simulink model "SIM_Overview"  (R2020b)
settings: Solver=FixedStepAuto  StartTime=0.0  StopTime=params.time.stop  FixedStep=1  RelTol=1e-3
PreLoadFcn:
  | run('sim_initial_values.m')
values from neighbouring files (symbols this model uses):
  data = get_scenario(1)    [sim_initial_values.m]
  solar = get_solar_from_file(data.Date(1),data.Date(end))    [sim_initial_values.m]
undefined symbols (not defined in the file or in its folder): days, params, seconds
libraries: mylib x5
settings Model: Creator=janluca  LastModifiedBy=janluca
settings DataIOCC: LimitDataPoints=on  MaxDataPoints=1

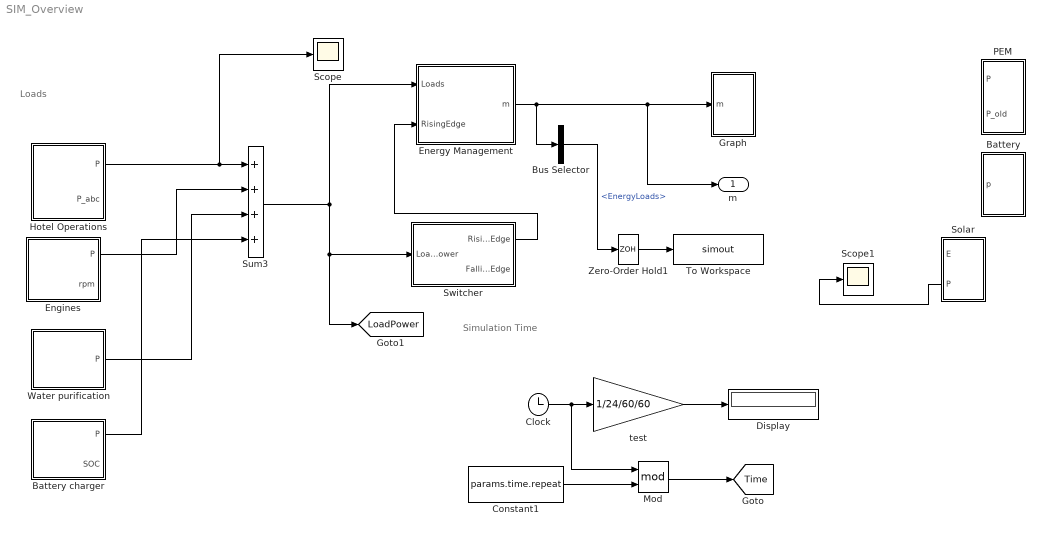
== system SIM_Overview ==
  note: Loads
  note: Simulation Time
  Battery : Subsystem
  Battery charger : Subsystem
  Bus Selector : BusSelector  OutputSignals=EnergyLoads
  Clock : Clock
      settings: Decimation=60000
  Constant1 : Constant  Value=params.time.repeat
  Display : Display
  Energy Management : Subsystem
  Engines : Subsystem
      mask Display: image('/Users/janluca/Projects/git/Masterthesis/MATLAB/icons/motor2.jpg'); % Use "Edit Image" on toolstrip to change.
  Graph : Subsystem
  Hotel Operations : Subsystem
      mask Display: image('/Users/janluca/Projects/git/Masterthesis/MATLAB/icons/bar.jpg'); % Use "Edit Image" on toolstrip to change.
  Mod : Math  Operator=mod  OutMin=[1]  OutMax=[3600]  SaturateOnIntegerOverflow=on
  PEM : Subsystem
  Scope : Scope
  Scope1 : Scope
  Solar : Subsystem
  Sum3 : Sum  Inputs=4
  Switcher : Subsystem
  To Workspace : ToWorkspace  VariableName=simout  SaveFormat=Timeseries  SampleTime=-1
  Water purification : Subsystem
      mask Display: image('/Users/janluca/Projects/git/Masterthesis/MATLAB/icons/wasserhahn.jpg'); % Use "Edit Image" on toolstrip to change.
  Zero-Order Hold1 : ZeroOrderHold  SampleTime=seconds(days(1))
  test : Gain  Gain=1/24/60/60
  m : Outport
  tag scope: LoadPower=global, Time=global
  wires:
  test/1 -> Display/1
  Constant1/1 -> Mod/2
  Mod/1 -> [Time]
  Clock/1 -> test/1, Mod/1
  Switcher/1(RisingEdge) -> Energy Management/2(RisingEdge)
  Energy Management/1(m) -> Bus Selector/1, m/1, Graph/1(m)
  Hotel Operations/1(P) -> Scope/1, Sum3/1
  Engines/1(P) -> Sum3/2
  Water purification/1(P) -> Sum3/3
  Battery charger/1(P) -> Sum3/4
  Sum3/1 -> [LoadPower], Switcher/1(LoadPower), Energy Management/1(Loads)
  Solar/2(P) -> Scope1/1
  Zero-Order Hold1/1 -> To Workspace/1
  Bus Selector/1 -> Zero-Order Hold1/1  "<EnergyLoads>"

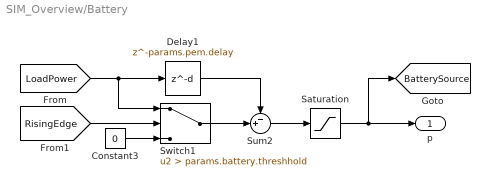
== system SIM_Overview/Battery ==
  Constant3 : Constant  Value=0
  Delay1 : Delay  DelayLength=params.pem.delay
  Saturation : Saturate  UpperLimit=params.battery.power  LowerLimit=0
  Sum2 : Sum  Inputs=-+|
  Switch1 : Switch  Criteria=u2 > Threshold  Threshold=params.battery.threshhold
  p : Outport
  tag scope: BatterySource=global
  wires:
  Constant3/1 -> Switch1/3
  Delay1/1 -> Sum2/1
  [LoadPower] -> Switch1/1, Delay1/1
  Sum2/1 -> Saturation/1
  Saturation/1 -> [BatterySource], p/1
  Switch1/1 -> Sum2/2
  [RisingEdge] -> Switch1/2

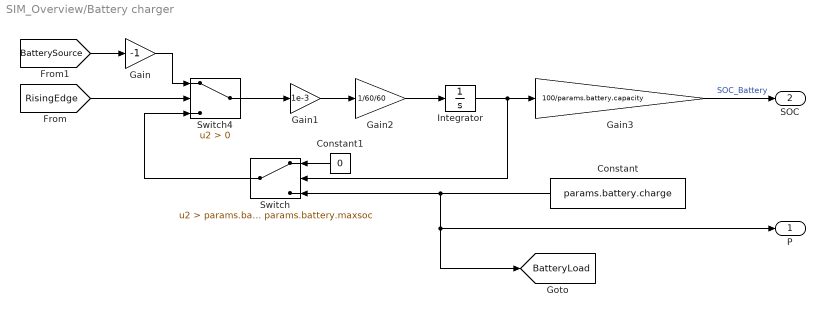
== system SIM_Overview/Battery charger ==
  Constant : Constant  Value=params.battery.charge
  Constant1 : Constant  Value=0
  Gain : Gain  Gain=-1
  Gain1 : Gain  Gain=1e-3
  Gain2 : Gain  Gain=1/60/60
  Gain3 : Gain  Gain=100/params.battery.capacity
  Integrator : Integrator  InitialCondition=params.battery.capacity * params.battery.initsoc
  Switch : Switch  Criteria=u2 > Threshold  Threshold=params.battery.capacity * params.battery.maxsoc
  Switch4 : Switch  Criteria=u2 > Threshold
  P : Outport
  SOC : Outport  Port=2
  tag scope: BatteryLoad=global
  wires:
  Gain1/1 -> Gain2/1
  Constant/1 -> P/1, [BatteryLoad], Switch/3
  Integrator/1 -> Switch/2, Gain3/1
  Gain/1 -> Switch4/1
  Gain2/1 -> Integrator/1
  Constant1/1 -> Switch/1
  Switch4/1 -> Gain1/1
  Switch/1 -> Switch4/3
  Gain3/1 -> SOC/1  "SOC_Battery"
  [RisingEdge] -> Switch4/2
  [BatterySource] -> Gain/1

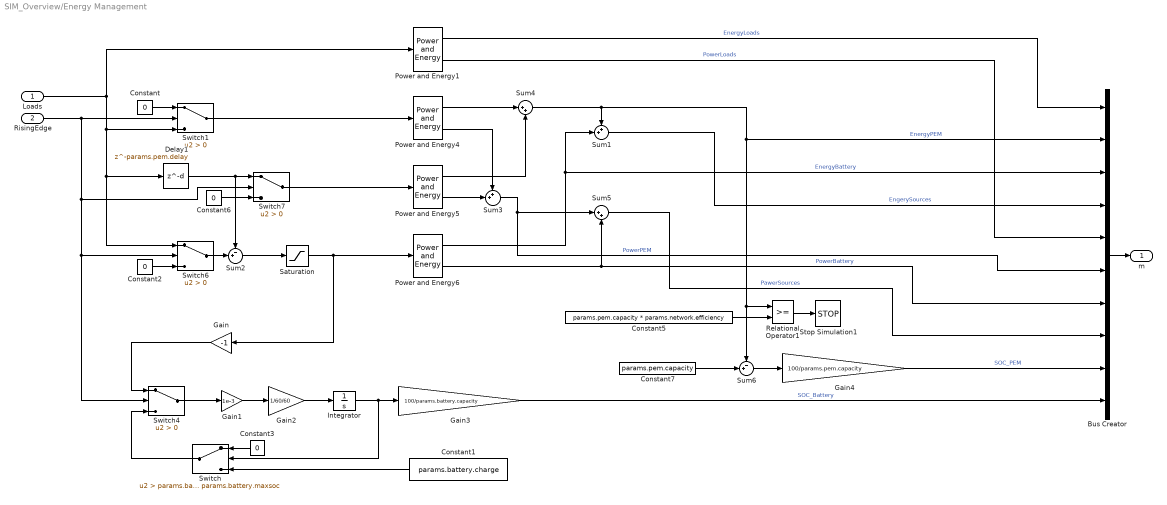
== system SIM_Overview/Energy Management ==
  Loads : Inport
  RisingEdge : Inport  Port=2
  Bus Creator : BusCreator  Inputs=10
  Constant{,2..3,6} (4 alike) : Constant  Value=0
  Constant1 : Constant  Value=params.battery.charge
  Constant5 : Constant  Value=params.pem.capacity * params.network.efficiency
  Constant7 : Constant  Value=params.pem.capacity
  Delay1 : Delay  DelayLength=params.pem.delay
  Gain : Gain  Gain=-1
  Gain1 : Gain  Gain=1e-3
  Gain2 : Gain  Gain=1/60/60
  Gain3 : Gain  Gain=100/params.battery.capacity
  Gain4 : Gain  Gain=100/params.pem.capacity
  Integrator : Integrator  InitialCondition=params.battery.capacity * params.battery.initsoc
  Power and Energy{1,4..6} (4 alike) : mylib/Power and Energy  SystemSampleTime=-1  VariantActivationTime=update diagram  Latency=0  AutoFrameSizeCalculation=off
  Relational Operator1 : RelationalOperator  OutDataTypeStr=boolean  RndMeth=Simplest
  Saturation : Saturate  UpperLimit=inf  LowerLimit=0
  Stop Simulation1 : Stop
  Sum1 : Sum  Inputs=++|
  Sum2 : Sum  Inputs=-+|
  Sum3 : Sum  Inputs=++|
  Sum4 : Sum  Inputs=|++
  Sum5 : Sum  Inputs=|++
  Sum6 : Sum  Inputs=-+|
  Switch : Switch  Criteria=u2 > Threshold  Threshold=params.battery.capacity * params.battery.maxsoc
  Switch{1,4,6..7} (4 alike) : Switch  Criteria=u2 > Threshold
  m : Outport
  wires:
  Loads/1 -> Switch6/1, Delay1/1, Switch1/3, Power and Energy1/1
  Constant/1 -> Switch1/1
  Constant2/1 -> Switch6/3
  Switch1/1 -> Power and Energy4/1
  Switch6/1 -> Sum2/2
  Sum2/1 -> Saturation/1
  Delay1/1 -> Sum2/1, Switch7/1
  Switch7/1 -> Power and Energy5/1
  Constant6/1 -> Switch7/3
  Power and Energy4/1 -> Sum4/1
  Power and Energy5/1 -> Sum4/2
  Sum4/1 -> Sum1/1, Bus Creator/2, Relational Operator1/1, Sum6/1  "EnergyPEM"
  Constant5/1 -> Relational Operator1/2
  Relational Operator1/1 -> Stop Simulation1/1
  Power and Energy6/1 -> Sum1/2, Bus Creator/3  "EnergyBattery"
  Sum1/1 -> Bus Creator/4  "EngerySources"
  Power and Energy5/2 -> Sum3/2
  Power and Energy4/2 -> Sum3/1
  Sum3/1 -> Bus Creator/6, Sum5/1  "PowerPEM"
  Sum5/1 -> Bus Creator/8  "PawerSources"
  Power and Energy6/2 -> Sum5/2, Bus Creator/7  "PowerBattery"
  Sum6/1 -> Gain4/1
  Constant7/1 -> Sum6/2
  Power and Energy1/1 -> Bus Creator/1  "EnergyLoads"
  Power and Energy1/2 -> Bus Creator/5  "PowerLoads"
  Gain4/1 -> Bus Creator/9  "SOC_PEM"
  Bus Creator/1 -> m/1
  Gain3/1 -> Bus Creator/10  "SOC_Battery"
  Gain2/1 -> Integrator/1
  Constant1/1 -> Switch/3
  Switch/1 -> Switch4/3
  Constant3/1 -> Switch/1
  Switch4/1 -> Gain1/1
  Gain/1 -> Switch4/1
  Gain1/1 -> Gain2/1
  RisingEdge/1 -> Switch4/2, Switch6/2, Switch7/2, Switch1/2
  Integrator/1 -> Switch/2, Gain3/1
  Saturation/1 -> Gain/1, Power and Energy6/1

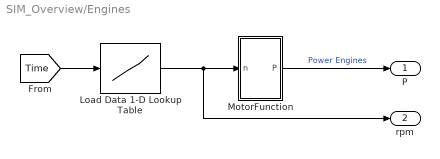
== system SIM_Overview/Engines ==
  Load Data 1-D Lookup Table : Lookup_n-D  NumberOfTableDimensions=1  BreakpointsForDimension1=data.time  BeginIndexSearchUsingPreviousIndexResult=on  Table=data.rpm  InternalRulePriority=Speed  RndMeth=Simplest  InputSameDT=on
  MotorFunction : Subsystem
  P : Outport
  rpm : Outport  Port=2
  wires:
  Load Data 1-D Lookup Table/1 -> rpm/1, MotorFunction/1(n)
  MotorFunction/1(P) -> P/1  "Power Engines"
  [Time] -> Load Data 1-D Lookup Table/1

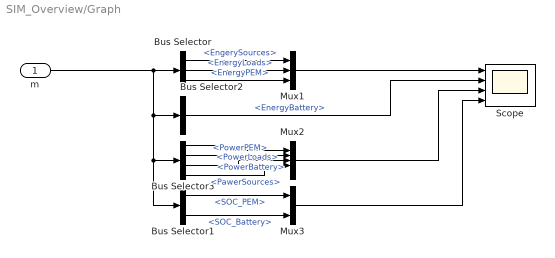
== system SIM_Overview/Graph ==
  m : Inport
  Bus Selector : BusSelector  OutputSignals=EngerySources,EnergyLoads,EnergyPEM
  Bus Selector1 : BusSelector  OutputSignals=SOC_PEM,SOC_Battery
  Bus Selector2 : BusSelector  OutputSignals=EnergyBattery
  Bus Selector3 : BusSelector  OutputSignals=PowerLoads,PowerPEM,PowerBattery,PawerSources
  Mux1 : Mux  Inputs=3
  Mux2 : Mux  Inputs=5
  Mux3 : Mux  Inputs=2
  Scope : Scope  NumInputPorts=4
  wires:
  m/1 -> Bus Selector2/1, Bus Selector3/1, Bus Selector1/1, Bus Selector/1
  Mux1/1 -> Scope/1
  Bus Selector2/1 -> Scope/2  "<EnergyBattery>"
  Bus Selector/2 -> Mux1/2  "<EnergyLoads>"
  Bus Selector3/4 -> Mux2/4  "<PawerSources>"
  Mux2/1 -> Scope/3
  Bus Selector3/3 -> Mux2/3  "<PowerBattery>"
  Bus Selector1/1 -> Mux3/1  "<SOC_PEM>"
  Bus Selector/3 -> Mux1/3  "<EnergyPEM>"
  Bus Selector3/2 -> Mux2/2  "<PowerPEM>"
  Bus Selector1/2 -> Mux3/2  "<SOC_Battery>"
  Mux3/1 -> Scope/4
  Bus Selector/1 -> Mux1/1  "<EngerySources>"
  Bus Selector3/1 -> Mux2/1  "<PowerLoads>"

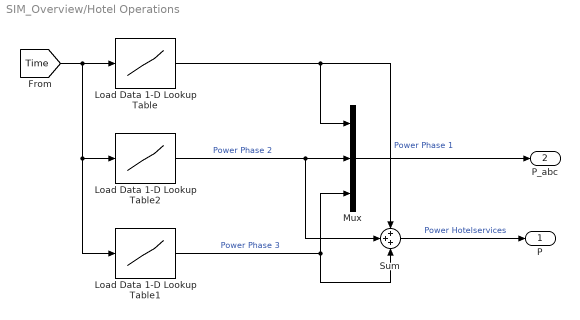
== system SIM_Overview/Hotel Operations ==
  Load Data 1-D Lookup Table : Lookup_n-D  NumberOfTableDimensions=1  BreakpointsForDimension1=data.time  BeginIndexSearchUsingPreviousIndexResult=on  Table=data.P11min  InternalRulePriority=Speed  RndMeth=Simplest  InputSameDT=on
  Load Data 1-D Lookup Table1 : Lookup_n-D  NumberOfTableDimensions=1  BreakpointsForDimension1=data.time  BeginIndexSearchUsingPreviousIndexResult=on  Table=data.P31min  InternalRulePriority=Speed  RndMeth=Simplest  InputSameDT=on
  Load Data 1-D Lookup Table2 : Lookup_n-D  NumberOfTableDimensions=1  BreakpointsForDimension1=data.time  BeginIndexSearchUsingPreviousIndexResult=on  Table=data.P21min  InternalRulePriority=Speed  RndMeth=Simplest  InputSameDT=on
  Mux : Mux  Inputs=3
  Sum : Sum  Inputs=+++
  P : Outport
  P_abc : Outport  Port=2
  wires:
  Load Data 1-D Lookup Table/1 -> Mux/1, Sum/1  "Power Phase 1"
  Load Data 1-D Lookup Table2/1 -> Sum/2, Mux/2  "Power Phase 2"
  Load Data 1-D Lookup Table1/1 -> Sum/3, Mux/3  "Power Phase 3"
  Mux/1 -> P_abc/1
  [Time] -> Load Data 1-D Lookup Table1/1, Load Data 1-D Lookup Table2/1, Load Data 1-D Lookup Table/1
  Sum/1 -> P/1  "Power Hotelservices"

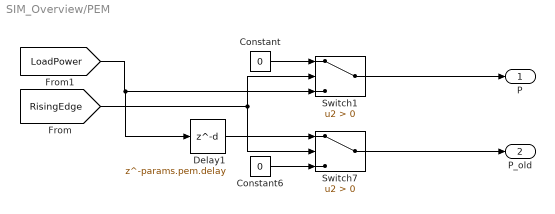
== system SIM_Overview/PEM ==
  Constant : Constant  Value=0
  Constant6 : Constant  Value=0
  Delay1 : Delay  DelayLength=params.pem.delay
  Switch1 : Switch  Criteria=u2 > Threshold
  Switch7 : Switch  Criteria=u2 > Threshold
  P : Outport
  P_old : Outport  Port=2
  wires:
  Switch1/1 -> P/1
  [RisingEdge] -> Switch1/2, Switch7/2
  Constant6/1 -> Switch7/3
  [LoadPower] -> Delay1/1, Switch1/3
  Delay1/1 -> Switch7/1
  Constant/1 -> Switch1/1
  Switch7/1 -> P_old/1

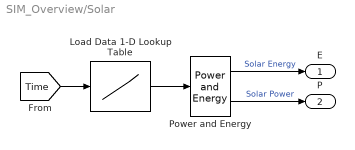
== system SIM_Overview/Solar ==
  Load Data 1-D Lookup Table : Lookup_n-D  NumberOfTableDimensions=1  BreakpointsForDimension1=solar.time  BeginIndexSearchUsingPreviousIndexResult=on  Table=solar.power  InternalRulePriority=Speed  RndMeth=Simplest  InputSameDT=on
  Power and Energy : mylib/Power and Energy  SystemSampleTime=-1  VariantActivationTime=update diagram  Latency=0  AutoFrameSizeCalculation=off
  E : Outport
  P : Outport  Port=2
  wires:
  Power and Energy/2 -> P/1  "Solar Power"
  Power and Energy/1 -> E/1  "Solar Energy"
  [Time] -> Load Data 1-D Lookup Table/1
  Load Data 1-D Lookup Table/1 -> Power and Energy/1

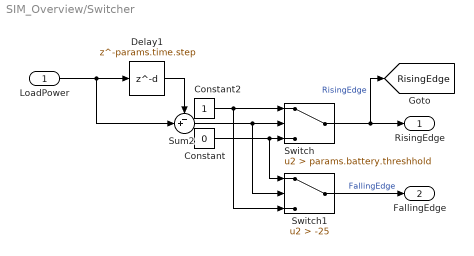
== system SIM_Overview/Switcher ==
  LoadPower : Inport
  Constant : Constant  Value=0
  Constant2 : Constant
  Delay1 : Delay  DelayLength=params.time.step
  Sum2 : Sum  Inputs=-+|
  Switch : Switch  Criteria=u2 > Threshold  Threshold=params.battery.threshhold
  Switch1 : Switch  Criteria=u2 > Threshold  Threshold=-25
  RisingEdge : Outport
  FallingEdge : Outport  Port=2
  tag scope: RisingEdge=global
  wires:
  Switch/1 -> [RisingEdge], RisingEdge/1  "RisingEdge"
  LoadPower/1 -> Sum2/2, Delay1/1
  Delay1/1 -> Sum2/1
  Constant/1 -> Switch1/1, Switch/3
  Switch1/1 -> FallingEdge/1  "FallingEdge"
  Constant2/1 -> Switch/1, Switch1/3
  Sum2/1 -> Switch/2, Switch1/2

== system SIM_Overview/Water purification ==
  Constant3 : Constant  Value=0.5e3
  P : Outport
  wires:
  Constant3/1 -> P/1  "Power water purification"

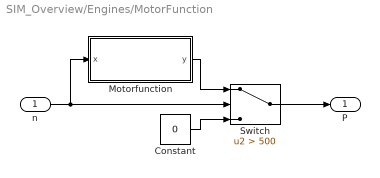
== system SIM_Overview/Engines/MotorFunction ==
  n : Inport
  Constant : Constant  Value=0
  Motorfunction : Subsystem  TreatAsAtomicUnit=on
  Switch : Switch  Criteria=u2 > Threshold  Threshold=500
  P : Outport
  wires:
  n/1 -> Switch/2, Motorfunction/1(x)
  Constant/1 -> Switch/3
  Motorfunction/1(y) -> Switch/1
  Switch/1 -> P/1

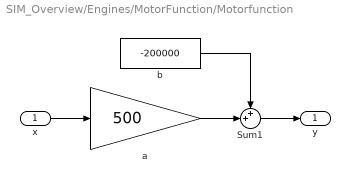
== system SIM_Overview/Engines/MotorFunction/Motorfunction ==
  x : Inport
  Sum1 : Sum  Inputs=++|
  a : Gain  Gain=500
  b : Constant  Value=-200000
  y : Outport
  wires:
  b/1 -> Sum1/1
  a/1 -> Sum1/2
  Sum1/1 -> y/1
  x/1 -> a/1
